simulink model "QuadrupedURDF"  (R2023b)
settings: Solver=VariableStepAuto  StartTime=0.0  StopTime=10.0  RelTol=1e-3
undefined symbols (not defined in the file or in its folder): body_mass, desired_speed, equilibrium_length, fixed_time, k_landing_angle, k_slip, kd, kp, lower_leg_length, max_torque, shin_mass, thigh_mass, upper_leg_length, X, x_contact, Y, y_contact, Z, z_contact
libraries: sm_lib x94, nesl_utility x21, slpidlib x10
(part 3 of 3)

== system QuadrupedURDF/Environment//Plant/Rear_Right_Thigh ==
  Inertia : sm_lib/Body Elements/Inertia  InertiaType=Custom  Mass=thigh_mass  MassUnits=kg  CenterOfMass=[0, 0, 0]  CenterOfMassUnits=m  MomentsOfInertia=[0.000703443703532356, 0.000379089863098611, 0.00102411507237722]  MomentsOfInertiaUnits=kg*m^2  ProductsOfInertia=[-1.02974442751944e-06, -1.25476848652012e-07, 5.05069776933996e-07]  ProductsOfInertiaUnits=kg*m^2  GraphicType=None  MarkerShape=Inertia  MarkerSize=20  GraphicVisPropType=SimpleVisualProperties  GraphicDiffuseColor=[0.5 0.5 0.5]  GraphicSpecularColor=[0.5 0.5 0.5 1.0]  GraphicAmbientColor=[0.15 0.15 0.15 1.0]  GraphicEmissiveColor=[0.0 0.0 0.0 1.0]  GraphicShininess=75  GraphicOpacity=1.0
  InertiaOriginTransform : sm_lib/Frames and Transforms/Rigid Transform  TranslationMethod=Cartesian  TranslationStandardOffset=0  TranslationStandardOffsetUnits=m  TranslationStandardAxis=+Z  TranslationCartesianOffset=[2.43741414215626e-05, -0.0142051404026354, -0.00547111407205259]  TranslationCartesianOffsetUnits=m  TranslationROffset=0  TranslationROffsetUnits=m  TranslationZOffset=0  TranslationZOffsetUnits=m  TranslationThetaOffset=0  TranslationThetaOffsetUnits=deg  RotationMethod=RotationSequence  RotationAngleUnits=deg  RotationStandardAxis=+Z  RotationAngle=0.0  RotationArbitraryAxis=[0 0 1]  FollAlignAxisA=+X  BaseAlignAxisA=+Y  FollAlignAxisB=+Y  BaseAlignAxisB=+Z  RotationSequenceAxes=BaseAxes  RotationSequence=XYZ  RotationSequenceAngles=[0, 0, 0]  RotationSequenceAnglesUnits=rad  RotationMatrix=[1 0 0; 0 1 0; 0 0 1]  Quaternion=[1 0 0 0]
  Rear_Right_Hip_AxisInvTransform : sm_lib/Frames and Transforms/Rigid Transform  TranslationMethod=Cartesian  TranslationStandardOffset=0  TranslationStandardOffsetUnits=m  TranslationStandardAxis=+Z  TranslationCartesianOffset=[0, 0, 0]  TranslationCartesianOffsetUnits=m  TranslationROffset=0  TranslationROffsetUnits=m  TranslationZOffset=0  TranslationZOffsetUnits=m  TranslationThetaOffset=0  TranslationThetaOffsetUnits=deg  RotationMethod=ArbitraryAxis  RotationAngleUnits=rad  RotationStandardAxis=+Z  RotationAngle=3.141592653589793  RotationArbitraryAxis=[1, 0, 0]  FollAlignAxisA=+X  BaseAlignAxisA=+Y  FollAlignAxisB=+Y  BaseAlignAxisB=+Z  RotationSequenceAxes=FollowerAxes  RotationSequence=XYX  RotationSequenceAngles=[0 0 0]  RotationSequenceAnglesUnits=deg  RotationMatrix=[1 0 0; 0 1 0; 0 0 1]  Quaternion=[1 0 0 0]
  Rear_Right_Knee_AxisTransform : sm_lib/Frames and Transforms/Rigid Transform  TranslationMethod=Cartesian  TranslationStandardOffset=0  TranslationStandardOffsetUnits=m  TranslationStandardAxis=+Z  TranslationCartesianOffset=[0, 0, 0]  TranslationCartesianOffsetUnits=m  TranslationROffset=0  TranslationROffsetUnits=m  TranslationZOffset=0  TranslationZOffsetUnits=m  TranslationThetaOffset=0  TranslationThetaOffsetUnits=deg  RotationMethod=ArbitraryAxis  RotationAngleUnits=rad  RotationStandardAxis=+Z  RotationAngle=0  RotationArbitraryAxis=[1, 0, 0]  FollAlignAxisA=+X  BaseAlignAxisA=+Y  FollAlignAxisB=+Y  BaseAlignAxisB=+Z  RotationSequenceAxes=FollowerAxes  RotationSequence=XYX  RotationSequenceAngles=[0 0 0]  RotationSequenceAnglesUnits=deg  RotationMatrix=[1 0 0; 0 1 0; 0 0 1]  Quaternion=[1 0 0 0]
  Rear_Right_Knee_OriginTransform : sm_lib/Frames and Transforms/Rigid Transform  TranslationMethod=Cartesian  TranslationStandardOffset=0  TranslationStandardOffsetUnits=m  TranslationStandardAxis=+Z  TranslationCartesianOffset=[0, -0.13624999987, 0.0151249999999999]  TranslationCartesianOffsetUnits=m  TranslationROffset=0  TranslationROffsetUnits=m  TranslationZOffset=0  TranslationZOffsetUnits=m  TranslationThetaOffset=0  TranslationThetaOffsetUnits=deg  RotationMethod=RotationSequence  RotationAngleUnits=deg  RotationStandardAxis=+Z  RotationAngle=0.0  RotationArbitraryAxis=[0 0 1]  FollAlignAxisA=+X  BaseAlignAxisA=+Y  FollAlignAxisB=+Y  BaseAlignAxisB=+Z  RotationSequenceAxes=BaseAxes  RotationSequence=XYZ  RotationSequenceAngles=[0, 0, 0]  RotationSequenceAnglesUnits=rad  RotationMatrix=[1 0 0; 0 1 0; 0 0 1]  Quaternion=[1 0 0 0]
  ReferenceFrame : sm_lib/Frames and Transforms/Reference Frame
  Visual : sm_lib/Body Elements/File Solid  ExtGeomFileName=Quadruped URDF/meshes/Rear Right Thigh.STL  UnitType=Custom  ExtGeomFileUnits=m  StepReaderType=HEX  ExportConvexHullGeometry=off  InertiaType=Custom  Mass=0  MassUnits=kg  CenterOfMass=[0, 0, 0]  CenterOfMassUnits=m  MomentsOfInertia=[0, 0, 0]  MomentsOfInertiaUnits=kg*m^2  ProductsOfInertia=[0, 0, 0]  ProductsOfInertiaUnits=kg*m^2  BasedOnType=DensityFromFile  Density=1000  DensityUnits=kg/m^3  DoExposeReferenceFrame=on  SerializedFrames=<Frames/>  GraphicType=FromGeometry  MarkerShape=Sphere  MarkerSize=10  GraphicVisPropType=SimpleVisualProperties  GraphicDiffuseColor=[1, 1, 1]  GraphicSpecularColor=[0.5 0.5 0.5 1.0]  GraphicAmbientColor=[0.15 0.15 0.15 1.0]  GraphicEmissiveColor=[0.0 0.0 0.0 1.0]  GraphicShininess=75  GraphicOpacity=1
  VisualOriginTransform : sm_lib/Frames and Transforms/Rigid Transform  TranslationMethod=Cartesian  TranslationStandardOffset=0  TranslationStandardOffsetUnits=m  TranslationStandardAxis=+Z  TranslationCartesianOffset=[0, 0, 0]  TranslationCartesianOffsetUnits=m  TranslationROffset=0  TranslationROffsetUnits=m  TranslationZOffset=0  TranslationZOffsetUnits=m  TranslationThetaOffset=0  TranslationThetaOffsetUnits=deg  RotationMethod=RotationSequence  RotationAngleUnits=deg  RotationStandardAxis=+Z  RotationAngle=0.0  RotationArbitraryAxis=[0 0 1]  FollAlignAxisA=+X  BaseAlignAxisA=+Y  FollAlignAxisB=+Y  BaseAlignAxisB=+Z  RotationSequenceAxes=BaseAxes  RotationSequence=XYZ  RotationSequenceAngles=[0, 0, 0]  RotationSequenceAnglesUnits=rad  RotationMatrix=[1 0 0; 0 1 0; 0 0 1]  Quaternion=[1 0 0 0]
  F : PMIOPort  Side=Left
  F1 : PMIOPort  Port=2  Side=Right
  connections:
  Inertia/RConn1 -- InertiaOriginTransform/RConn1
  Rear_Right_Hip_AxisInvTransform/RConn1 -- F/RConn1
  Rear_Right_Knee_AxisTransform/RConn1 -- F1/RConn1
  Rear_Right_Knee_AxisTransform/LConn1 -- Rear_Right_Knee_OriginTransform/RConn1
  Rear_Right_Hip_AxisInvTransform/LConn1 -- InertiaOriginTransform/LConn1 -- ReferenceFrame/RConn1 -- VisualOriginTransform/LConn1 -- Rear_Right_Knee_OriginTransform/LConn1
  Visual/RConn1 -- VisualOriginTransform/RConn1

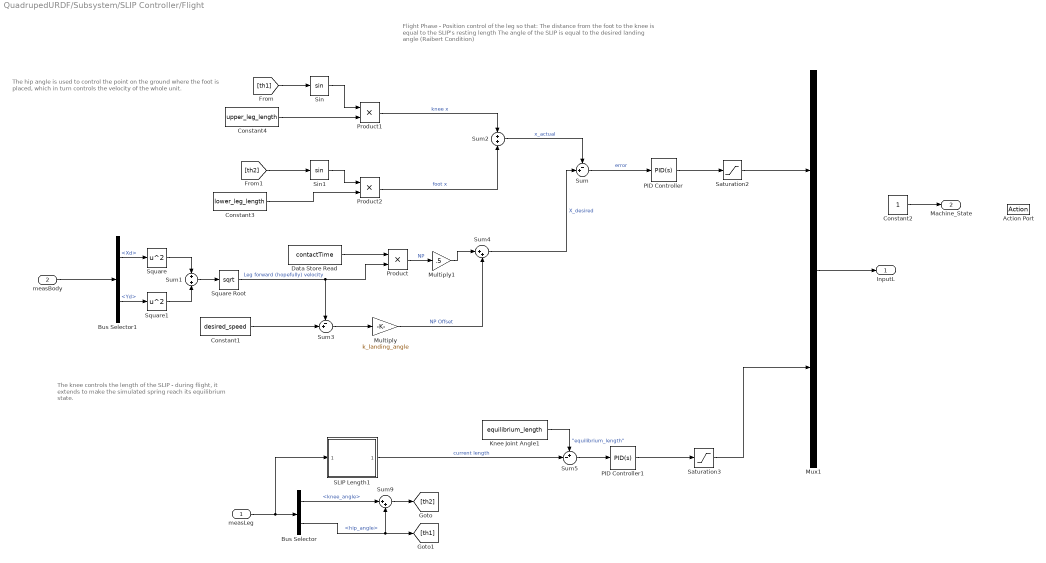
== system QuadrupedURDF/Subsystem/SLIP Controller/Flight ==
  note: Flight Phase - Position control of the leg so that:
      | The distance from the foot to the knee is equal to the SLIP's resting length
      | The angle of the SLIP is equal to the desired landing angle (Raibert Condition)
  note: The hip angle is used to control the point on the ground where the foot is
      | placed, which in turn controls the velocity of the whole unit.
  note: The knee controls the length of the SLIP - during flight, it
      | extends to make the simulated spring reach its equilibrium
      | state.
  measLeg : Inport
  measBody : Inport  Port=2
  Action Port : ActionPort
      settings: CopyFcn=Stateflow.SLINSF.SimulinkMan.removeBlockPreDeleteFcn  PreDeleteFcn=Stateflow.SLINSF.SimulinkMan.unsafePredeleteFcn
  Bus Selector : BusSelector  OutputSignals=knee_angle,hip_angle
  Bus Selector1 : BusSelector  OutputSignals=Xd,Yd
  Constant1 : Constant  Value=desired_speed
  Constant2 : Constant
  Constant3 : Constant  Value=lower_leg_length
  Constant4 : Constant  Value=upper_leg_length
  Data Store Read : DataStoreRead  DataStoreName=contactTime  IndexOptions=Index vector (dialog)  Indices=1  OutputSizes=1
  Knee Joint Angle1 : Constant  Value=equilibrium_length
  Multiply : Gain  Gain=k_landing_angle
  Multiply1 : Gain  Gain=.5
  Mux1 : Mux  Inputs=2
  PID Controller : slpidlib/PID Controller  Controller=PID  Form=Parallel  TimeDomain=Continuous-time  UseExternalTs=off  SampleTime=-1  IntegratorMethod=Forward Euler  FilterMethod=Forward Euler  ControllerParametersSource=internal  P=50  I=0  UseKiTs=off  D=10  N=100  UseFilter=on  TunerSelectOption=Transfer Function Based (PID Tuner App)  InitialConditionSource=internal  InitialConditionForIntegrator=0  InitialConditionForFilter=0  DifferentiatorICPrevScaledInput=0  ExternalReset=none  TrackingMode=off  Kt=1  LimitOutput=off  SatLimitsSource=internal  UpperSaturationLimit=inf  LowerSaturationLimit=-inf  LinearizeAsGain=on  AntiWindupMode=none  Kb=1  LimitIntegrator=off  UpperIntegratorSaturationLimit=inf  LowerIntegratorSaturationLimit=-inf  POutMin=[]  POutMax=[]  IOutMin=[]  IOutMax=[]  DOutMin=[]  DOutMax=[]  NOutMin=[]  NOutMax=[]  SumOutMin=[]  SumOutMax=[]  SaturationOutMin=[]  SaturationOutMax=[]  PParamMin=[]  PParamMax=[]  IParamMin=[]  IParamMax=[]  DParamMin=[]  DParamMax=[]  NParamMin=[]  NParamMax=[]  KbParamMin=[]  KbParamMax=[]  KtParamMin=[]  KtParamMax=[]  KbOutMin=[]  KbOutMax=[]  KtOutMin=[]  KtOutMax=[]  IntegratorOutMin=[]  IntegratorOutMax=[]  FilterOutMin=[]  FilterOutMax=[]  SumI1OutMin=[]  SumI1OutMax=[]  SumI2OutMin=[]  SumI2OutMax=[]  SumI3OutMin=[]  SumI3OutMax=[]  SumI4OutMin=[]  SumI4OutMax=[]  SumDOutMin=[]  SumDOutMax=[]  DifferentiatorOutMin=[]  DifferentiatorOutMax=[]  FilterDiffOutCoefMin=[]  FilterDiffOutCoefMax=[]  ReciprocalOutMin=[]  ReciprocalOutMax=[]  SumDenOutMin=[]  SumDenOutMax=[]  SumNumOutMin=[]  SumNumOutMax=[]  DivideOutMin=[]  DivideOutMax=[]  UdiffTsProdOutMin=[]  UdiffTsProdOutMax=[]  NTsProdOutMin=[]  NTsProdOutMax=[]  UintegralTsProdOutMin=[]  UintegralTsProdOutMax=[]  UngainTsProdOutMin=[]  UngainTsProdOutMax=[]  ClampingZeroOutDataTypeStr=Inherit: Inherit via back propagation  ClampingZeroOutMin=[]  ClampingZeroOutMax=[]  FilterDenConstantOutDataTypeStr=Inherit: Inherit via back propagation  FilterDenConstantOutMin=[]  FilterDenConstantOutMax=[]  PCopyOutDataTypeStr=Inherit: Inherit via back propagation  PCopyOutMin=[]  PCopyOutMax=[]  NCopyOutDataTypeStr=Inherit: Inherit via back propagation  NCopyOutMin=[]  NCopyOutMax=[]  IntegratorContinuousStateAttributes=''  IntegratorStateMustResolveToSignalObject=off  IntegratorRTWStateStorageClass=Auto  FilterContinuousStateAttributes=''  FilterStateMustResolveToSignalObject=off  FilterRTWStateStorageClass=Auto  ParallelPVariant=InternalParameters  IdealPVariant=Disabled  IVariant=InternalParameters  DVariant=InternalParameters  IntegratorVariant=Continuous  SatVariant=Disabled  AWVariant=Passthrough  PCopyVariant=Disabled  TRVariant=Disabled  FdbkBlocksVariant=Forward  IdealPFdbkVariant=Disabled  SatFdbkVariant=Disabled  DerivativeFilterVariant=ContFilter  NVariant=InternalParameters  NCopyVariant=Disabled  FilterICVariant=InternalICsFilter  IntegratorICVariant=InternalICs  ExternalResetVariant=Disabled  TRSumVariant=Passthrough  SumFdbkVariant=Disabled  SumVariant=Sum_PID  TsampFilterVariant=InternalTs  TsampNgainVariant=Passthrough  TsampIntegralVariant=Disabled_SignalSpec  ExternalSaturationOutDataTypeStr=Inherit: Same as second input
  PID Controller1 : slpidlib/PID Controller  Controller=PID  Form=Parallel  TimeDomain=Continuous-time  UseExternalTs=off  SampleTime=-1  IntegratorMethod=Forward Euler  FilterMethod=Forward Euler  ControllerParametersSource=internal  P=50  I=0  UseKiTs=off  D=5  N=100  UseFilter=on  TunerSelectOption=Transfer Function Based (PID Tuner App)  InitialConditionSource=internal  InitialConditionForIntegrator=0  InitialConditionForFilter=0  DifferentiatorICPrevScaledInput=0  ExternalReset=none  TrackingMode=off  Kt=1  LimitOutput=off  SatLimitsSource=internal  UpperSaturationLimit=inf  LowerSaturationLimit=-inf  LinearizeAsGain=on  AntiWindupMode=none  Kb=1  LimitIntegrator=off  UpperIntegratorSaturationLimit=inf  LowerIntegratorSaturationLimit=-inf  POutMin=[]  POutMax=[]  IOutMin=[]  IOutMax=[]  DOutMin=[]  DOutMax=[]  NOutMin=[]  NOutMax=[]  SumOutMin=[]  SumOutMax=[]  SaturationOutMin=[]  SaturationOutMax=[]  PParamMin=[]  PParamMax=[]  IParamMin=[]  IParamMax=[]  DParamMin=[]  DParamMax=[]  NParamMin=[]  NParamMax=[]  KbParamMin=[]  KbParamMax=[]  KtParamMin=[]  KtParamMax=[]  KbOutMin=[]  KbOutMax=[]  KtOutMin=[]  KtOutMax=[]  IntegratorOutMin=[]  IntegratorOutMax=[]  FilterOutMin=[]  FilterOutMax=[]  SumI1OutMin=[]  SumI1OutMax=[]  SumI2OutMin=[]  SumI2OutMax=[]  SumI3OutMin=[]  SumI3OutMax=[]  SumI4OutMin=[]  SumI4OutMax=[]  SumDOutMin=[]  SumDOutMax=[]  DifferentiatorOutMin=[]  DifferentiatorOutMax=[]  FilterDiffOutCoefMin=[]  FilterDiffOutCoefMax=[]  ReciprocalOutMin=[]  ReciprocalOutMax=[]  SumDenOutMin=[]  SumDenOutMax=[]  SumNumOutMin=[]  SumNumOutMax=[]  DivideOutMin=[]  DivideOutMax=[]  UdiffTsProdOutMin=[]  UdiffTsProdOutMax=[]  NTsProdOutMin=[]  NTsProdOutMax=[]  UintegralTsProdOutMin=[]  UintegralTsProdOutMax=[]  UngainTsProdOutMin=[]  UngainTsProdOutMax=[]  ClampingZeroOutDataTypeStr=Inherit: Inherit via back propagation  ClampingZeroOutMin=[]  ClampingZeroOutMax=[]  FilterDenConstantOutDataTypeStr=Inherit: Inherit via back propagation  FilterDenConstantOutMin=[]  FilterDenConstantOutMax=[]  PCopyOutDataTypeStr=Inherit: Inherit via back propagation  PCopyOutMin=[]  PCopyOutMax=[]  NCopyOutDataTypeStr=Inherit: Inherit via back propagation  NCopyOutMin=[]  NCopyOutMax=[]  IntegratorContinuousStateAttributes=''  IntegratorStateMustResolveToSignalObject=off  IntegratorRTWStateStorageClass=Auto  FilterContinuousStateAttributes=''  FilterStateMustResolveToSignalObject=off  FilterRTWStateStorageClass=Auto  ParallelPVariant=InternalParameters  IdealPVariant=Disabled  IVariant=InternalParameters  DVariant=InternalParameters  IntegratorVariant=Continuous  SatVariant=Disabled  AWVariant=Passthrough  PCopyVariant=Disabled  TRVariant=Disabled  FdbkBlocksVariant=Forward  IdealPFdbkVariant=Disabled  SatFdbkVariant=Disabled  DerivativeFilterVariant=ContFilter  NVariant=InternalParameters  NCopyVariant=Disabled  FilterICVariant=InternalICsFilter  IntegratorICVariant=InternalICs  ExternalResetVariant=Disabled  TRSumVariant=Passthrough  SumFdbkVariant=Disabled  SumVariant=Sum_PID  TsampFilterVariant=InternalTs  TsampNgainVariant=Passthrough  TsampIntegralVariant=Disabled_SignalSpec  ExternalSaturationOutDataTypeStr=Inherit: Same as second input
  Product : Product
  Product1 : Product
  Product2 : Product
  SLIP Length1 : Subsystem
  Saturation2 : Saturate  UpperLimit=max_torque  LowerLimit=-max_torque
  Saturation3 : Saturate  UpperLimit=max_torque  LowerLimit=-max_torque
  Sin : Trigonometry
  Sin1 : Trigonometry
  Square : Math  Operator=square
  Square Root : Sqrt
  Square1 : Math  Operator=square
  Sum : Sum  Inputs=-+|
  Sum1 : Sum  Inputs=+|+
  Sum2 : Sum  Inputs=+|+
  Sum3 : Sum  Inputs=-+|
  Sum4 : Sum  Inputs=|++
  Sum5 : Sum  Inputs=+-|
  Sum9 : Sum  Inputs=|++
  InputL : Outport
  Machine_State : Outport  Port=2
  wires:
  Sum1/1 -> Square Root/1
  Bus Selector1/2 -> Square1/1  "<Yd>"
  Product1/1 -> Sum2/1  "knee x"
  Sin1/1 -> Product2/1
  [th1] -> Sin/1
  Constant2/1 -> Machine_State/1
  Saturation3/1 -> Mux1/2
  Sum4/1 -> Sum/2  "X_desired"
  Knee Joint Angle1/1 -> Sum5/1  "\"equilibrium_length\""
  Multiply1/1 -> Sum4/1
  Constant1/1 -> Sum3/2
  Sin/1 -> Product1/1
  [th2] -> Sin1/1
  Sum5/1 -> PID Controller1/1
  PID Controller/1 -> Saturation2/1
  Bus Selector1/1 -> Square/1  "<Xd>"
  Data Store Read/1 -> Product/1
  Bus Selector/2 -> Sum9/2, [th1]  "<hip_angle>"
  Multiply/1 -> Sum4/2  "NP Offset"
  Sum9/1 -> [th2]
  Bus Selector/1 -> Sum9/1  "<knee_angle>"
  measLeg/1 -> SLIP Length1/1(measLeg), Bus Selector/1
  SLIP Length1/1(current length) -> Sum5/2  "current length"
  Square Root/1 -> Product/2, Sum3/1  "Leg forward (hopefully) velocity"
  PID Controller1/1 -> Saturation3/1
  Sum3/1 -> Multiply/1
  Saturation2/1 -> Mux1/1
  Mux1/1 -> InputL/1
  Constant4/1 -> Product1/2
  Sum/1 -> PID Controller/1  "error"
  Sum2/1 -> Sum/1  "x_actual"
  Product2/1 -> Sum2/2  "foot x"
  Product/1 -> Multiply1/1  "NP"
  Constant3/1 -> Product2/2
  Square1/1 -> Sum1/2
  Square/1 -> Sum1/1
  measBody/1 -> Bus Selector1/1

== system QuadrupedURDF/Subsystem/SLIP Controller/Stance ==
  note: Stance Phase - the SLIP is allowed to dictate the reaction of the leg
  measLeg : Inport
  Action Port : ActionPort
      settings: CopyFcn=Stateflow.SLINSF.SimulinkMan.removeBlockPreDeleteFcn  PreDeleteFcn=Stateflow.SLINSF.SimulinkMan.unsafePredeleteFcn
  Constant2 : Constant  Value=3
  Hip Torque Calculation : Subsystem
  Knee Torque Calculation : Subsystem
  Mux : Mux  Inputs=2
  Saturation : Saturate  UpperLimit=max_torque  LowerLimit=-max_torque
  Saturation1 : Saturate  UpperLimit=max_torque  LowerLimit=-max_torque
  InputL : Outport
  Machine_State : Outport  Port=2
  wires:
  Mux/1 -> InputL/1
  Constant2/1 -> Machine_State/1
  Knee Torque Calculation/1(knee torque) -> Saturation1/1  "knee torque unsat"
  Saturation/1 -> Mux/1  "hip torque sat"
  Saturation1/1 -> Mux/2  "knee torque sat"
  Hip Torque Calculation/1(hip torque) -> Knee Torque Calculation/1(hip torque), Saturation/1  "hip torque unsat"
  measLeg/1 -> Hip Torque Calculation/1(measLeg), Knee Torque Calculation/2(measLeg)

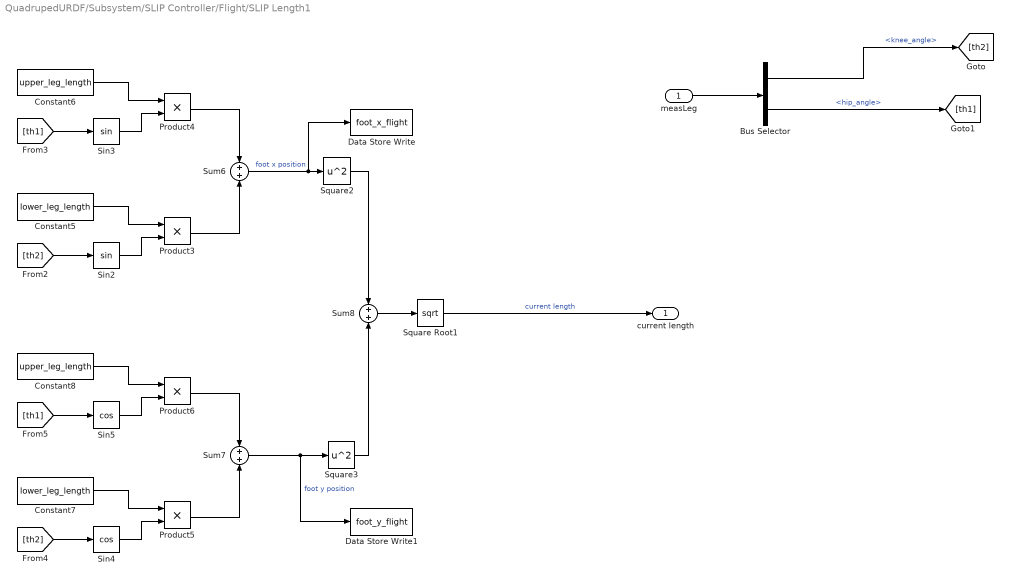
== system QuadrupedURDF/Subsystem/SLIP Controller/Flight/SLIP Length1 ==
  measLeg : Inport
  Bus Selector : BusSelector  OutputSignals=knee_angle,hip_angle
  Constant5 : Constant  Value=lower_leg_length
  Constant6 : Constant  Value=upper_leg_length
  Constant7 : Constant  Value=lower_leg_length
  Constant8 : Constant  Value=upper_leg_length
  Data Store Write : DataStoreWrite  DataStoreName=foot_x_flight  IndexOptions=Index vector (dialog)  Indices=1  OutputSizes=1
  Data Store Write1 : DataStoreWrite  DataStoreName=foot_y_flight  IndexOptions=Index vector (dialog)  Indices=1  OutputSizes=1
  Product{3..6} (4 alike) : Product
  Sin2 : Trigonometry
  Sin3 : Trigonometry
  Sin4 : Trigonometry  Operator=cos
  Sin5 : Trigonometry  Operator=cos
  Square Root1 : Sqrt
  Square2 : Math  Operator=square
  Square3 : Math  Operator=square
  Sum6 : Sum  Inputs=+|+
  Sum7 : Sum  Inputs=+|+
  Sum8 : Sum  Inputs=+|+
  current length : Outport
  wires:
  Square2/1 -> Sum8/1
  Sum7/1 -> Data Store Write1/1, Square3/1  "foot y position"
  [th2] -> Sin2/1
  Square3/1 -> Sum8/2
  Sin4/1 -> Product5/2
  Constant5/1 -> Product3/1
  Constant7/1 -> Product5/1
  Product6/1 -> Sum7/1
  Product3/1 -> Sum6/2
  [th2] -> Sin4/1
  Product5/1 -> Sum7/2
  [th1] -> Sin5/1
  Sin3/1 -> Product4/2
  Constant8/1 -> Product6/1
  Sin5/1 -> Product6/2
  Sin2/1 -> Product3/2
  Sum6/1 -> Data Store Write/1, Square2/1  "foot x position"
  Constant6/1 -> Product4/1
  Product4/1 -> Sum6/1
  Sum8/1 -> Square Root1/1
  [th1] -> Sin3/1
  Square Root1/1 -> current length/1  "current length"
  Bus Selector/1 -> [th2]  "<knee_angle>"
  Bus Selector/2 -> [th1]  "<hip_angle>"
  measLeg/1 -> Bus Selector/1

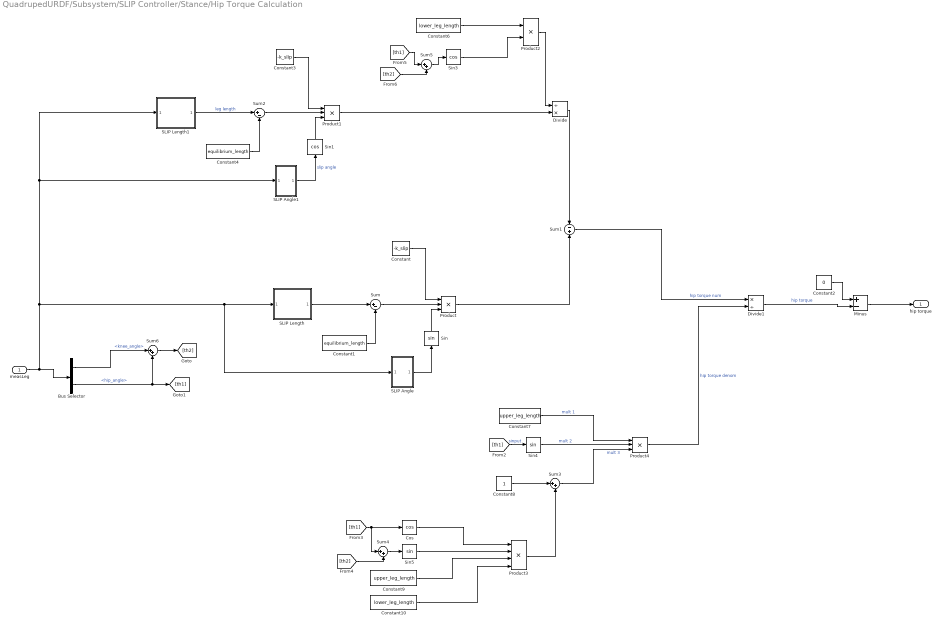
== system QuadrupedURDF/Subsystem/SLIP Controller/Stance/Hip Torque Calculation ==
  measLeg : Inport
  Bus Selector : BusSelector  OutputSignals=knee_angle,hip_angle
  Constant : Constant  Value=-k_slip
  Constant1 : Constant  Value=equilibrium_length
  Constant10 : Constant  Value=lower_leg_length
  Constant2 : Constant  Value=0
  Constant3 : Constant  Value=-k_slip
  Constant4 : Constant  Value=equilibrium_length
  Constant6 : Constant  Value=lower_leg_length
  Constant7 : Constant  Value=upper_leg_length
  Constant8 : Constant
  Constant9 : Constant  Value=upper_leg_length
  Cos : Trigonometry  Operator=cos
  Divide : Product  Inputs=/*
  Divide1 : Product  Inputs=*/
  Minus : Sum  Inputs=+-
  Product : Product  Inputs=3
  Product1 : Product  Inputs=3
  Product2 : Product
  Product3 : Product  Inputs=4
  Product4 : Product  Inputs=3
  SLIP Angle : Subsystem
  SLIP Angle1 : Subsystem
  SLIP Length : Subsystem
  SLIP Length1 : Subsystem
  Sin : Trigonometry
  Sin1 : Trigonometry  Operator=cos
  Sin3 : Trigonometry  Operator=cos
  Sin4 : Trigonometry
  Sin5 : Trigonometry
  Sum : Sum  Inputs=|+-
  Sum1 : Sum  Inputs=-|+
  Sum2 : Sum  Inputs=|+-
  Sum{3..6} (4 alike) : Sum  Inputs=|++
  hip torque : Outport
  wires:
  Sin1/1 -> Product1/3
  [th2] -> Sum4/2
  Constant/1 -> Product/1
  Sin5/1 -> Product3/2
  Constant7/1 -> Product4/1  "mult 1"
  Constant1/1 -> Sum/2
  Product2/1 -> Divide/1
  Product/1 -> Sum1/2
  Sin/1 -> Product/3
  Constant6/1 -> Product2/1
  Constant9/1 -> Product3/3
  Sum/1 -> Product/2
  Product3/1 -> Sum3/2
  Constant10/1 -> Product3/4
  SLIP Angle/1(Out1) -> Sin/1
  Sum1/1 -> Divide1/1  "hip torque num"
  Sum2/1 -> Product1/2
  Product4/1 -> Divide1/2  "hip torque denom"
  SLIP Length1/1(current length) -> Sum2/1  "leg length"
  Constant4/1 -> Sum2/2
  SLIP Angle1/1(Out1) -> Sin1/1  "slip angle"
  Divide1/1 -> Minus/2  "hip torque"
  Constant3/1 -> Product1/1
  Product1/1 -> Divide/2
  [th1] -> Sum4/1, Cos/1
  Sin3/1 -> Product2/2
  Sin4/1 -> Product4/2  "mult 2"
  Divide/1 -> Sum1/1
  SLIP Length/1(current length) -> Sum/1
  Sum3/1 -> Product4/3  "mult 3"
  [th1] -> Sin4/1  "sinput"
  Constant8/1 -> Sum3/1
  Cos/1 -> Product3/1
  Constant2/1 -> Minus/1
  Minus/1 -> hip torque/1
  Sum4/1 -> Sin5/1
  [th1] -> Sum5/1
  [th2] -> Sum5/2
  Sum5/1 -> Sin3/1
  measLeg/1 -> Bus Selector/1, SLIP Angle/1(measLeg), SLIP Length/1(measLeg), SLIP Angle1/1(measLeg), SLIP Length1/1(measLeg)
  Bus Selector/1 -> Sum6/1  "<knee_angle>"
  Bus Selector/2 -> Sum6/2, [th1]  "<hip_angle>"
  Sum6/1 -> [th2]

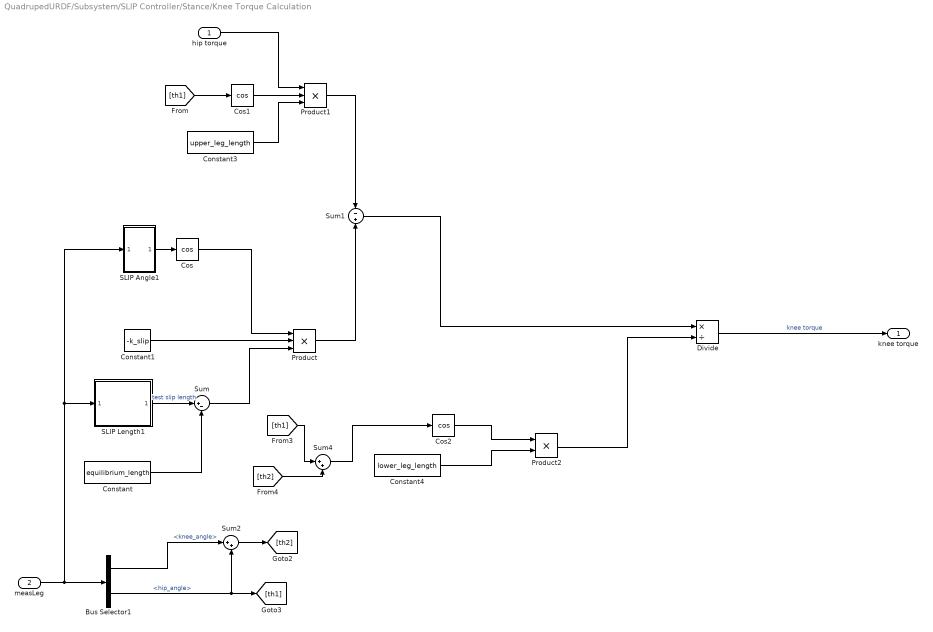
== system QuadrupedURDF/Subsystem/SLIP Controller/Stance/Knee Torque Calculation ==
  hip torque : Inport
  measLeg : Inport  Port=2
  Bus Selector1 : BusSelector  OutputSignals=knee_angle,hip_angle
  Constant : Constant  Value=equilibrium_length
  Constant1 : Constant  Value=-k_slip
  Constant3 : Constant  Value=upper_leg_length
  Constant4 : Constant  Value=lower_leg_length
  Cos : Trigonometry  Operator=cos
  Cos1 : Trigonometry  Operator=cos
  Cos2 : Trigonometry  Operator=cos
  Divide : Product  Inputs=*/
  Product : Product  Inputs=3
  Product1 : Product  Inputs=3
  Product2 : Product
  SLIP Angle1 : Subsystem
  SLIP Length1 : Subsystem
  Sum : Sum  Inputs=|+-
  Sum1 : Sum  Inputs=-|+
  Sum2 : Sum  Inputs=|++
  Sum4 : Sum  Inputs=|++
  knee torque : Outport
  wires:
  Constant3/1 -> Product1/3
  Constant/1 -> Sum/2
  Cos/1 -> Product/1
  Cos2/1 -> Product2/1
  SLIP Length1/1(current length) -> Sum/1  "test slip length"
  Sum1/1 -> Divide/1
  Constant4/1 -> Product2/2
  Product1/1 -> Sum1/1
  Constant1/1 -> Product/2
  [th1] -> Cos1/1
  Sum4/1 -> Cos2/1
  Cos1/1 -> Product1/2
  Product/1 -> Sum1/2
  SLIP Angle1/1(Out1) -> Cos/1
  Sum/1 -> Product/3
  Product2/1 -> Divide/2
  Divide/1 -> knee torque/1  "knee torque"
  hip torque/1 -> Product1/1
  [th1] -> Sum4/1
  [th2] -> Sum4/2
  measLeg/1 -> Bus Selector1/1, SLIP Length1/1(measLeg), SLIP Angle1/1(measLeg)
  Bus Selector1/1 -> Sum2/1  "<knee_angle>"
  Bus Selector1/2 -> Sum2/2, [th1]  "<hip_angle>"
  Sum2/1 -> [th2]

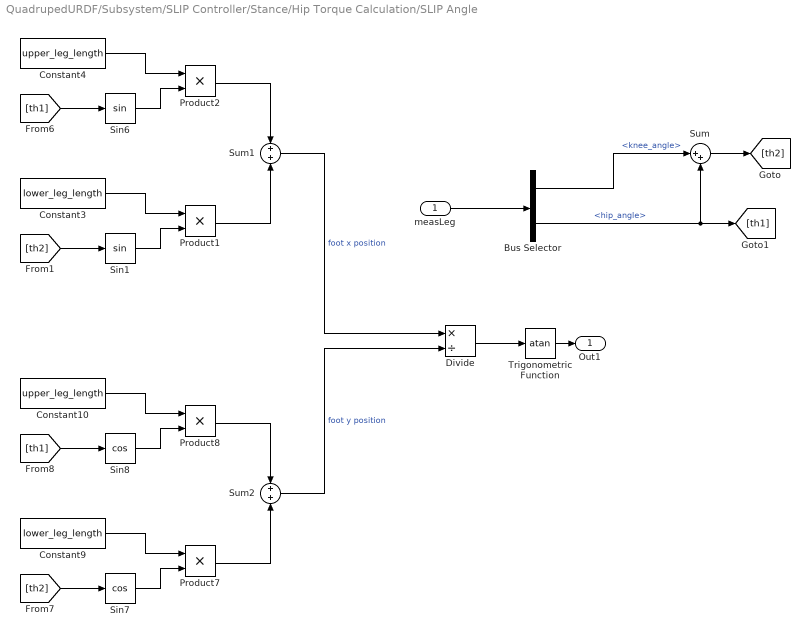
== system QuadrupedURDF/Subsystem/SLIP Controller/Stance/Hip Torque Calculation/SLIP Angle ==
  measLeg : Inport
  Bus Selector : BusSelector  OutputSignals=knee_angle,hip_angle
  Constant10 : Constant  Value=upper_leg_length
  Constant3 : Constant  Value=lower_leg_length
  Constant4 : Constant  Value=upper_leg_length
  Constant9 : Constant  Value=lower_leg_length
  Divide : Product  Inputs=*/
  Product{1..2,7..8} (4 alike) : Product
  Sin1 : Trigonometry
  Sin6 : Trigonometry
  Sin7 : Trigonometry  Operator=cos
  Sin8 : Trigonometry  Operator=cos
  Sum : Sum  Inputs=|++
  Sum1 : Sum  Inputs=+|+
  Sum2 : Sum  Inputs=+|+
  Trigonometric Function : Trigonometry  Operator=atan
  Out1 : Outport
  wires:
  Product2/1 -> Sum1/1
  Constant9/1 -> Product7/1
  Sin7/1 -> Product7/2
  Constant10/1 -> Product8/1
  Sin1/1 -> Product1/2
  [th1] -> Sin8/1
  Sin8/1 -> Product8/2
  Product7/1 -> Sum2/2
  [th2] -> Sin7/1
  Sum2/1 -> Divide/2  "foot y position"
  Trigonometric Function/1 -> Out1/1
  Product8/1 -> Sum2/1
  Sum1/1 -> Divide/1  "foot x position"
  Divide/1 -> Trigonometric Function/1
  [th1] -> Sin6/1
  Sin6/1 -> Product2/2
  [th2] -> Sin1/1
  Constant3/1 -> Product1/1
  Constant4/1 -> Product2/1
  Product1/1 -> Sum1/2
  Bus Selector/1 -> Sum/1  "<knee_angle>"
  Bus Selector/2 -> Sum/2, [th1]  "<hip_angle>"
  measLeg/1 -> Bus Selector/1
  Sum/1 -> [th2]

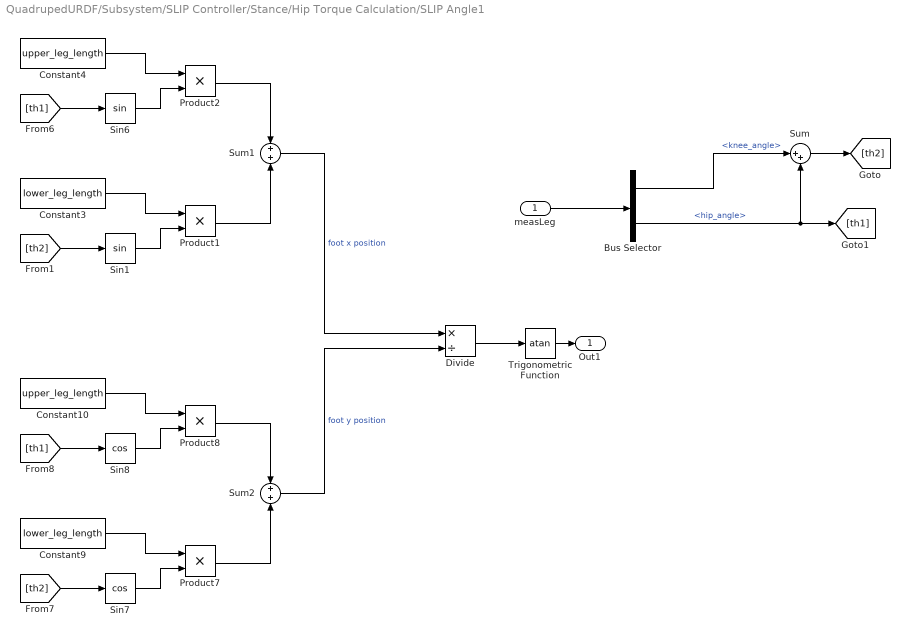
== system QuadrupedURDF/Subsystem/SLIP Controller/Stance/Hip Torque Calculation/SLIP Angle1 ==
  measLeg : Inport
  Bus Selector : BusSelector  OutputSignals=knee_angle,hip_angle
  Constant10 : Constant  Value=upper_leg_length
  Constant3 : Constant  Value=lower_leg_length
  Constant4 : Constant  Value=upper_leg_length
  Constant9 : Constant  Value=lower_leg_length
  Divide : Product  Inputs=*/
  Product{1..2,7..8} (4 alike) : Product
  Sin1 : Trigonometry
  Sin6 : Trigonometry
  Sin7 : Trigonometry  Operator=cos
  Sin8 : Trigonometry  Operator=cos
  Sum : Sum  Inputs=|++
  Sum1 : Sum  Inputs=+|+
  Sum2 : Sum  Inputs=+|+
  Trigonometric Function : Trigonometry  Operator=atan
  Out1 : Outport
  wires:
  Product2/1 -> Sum1/1
  Constant9/1 -> Product7/1
  Sin7/1 -> Product7/2
  Constant10/1 -> Product8/1
  Sin1/1 -> Product1/2
  [th1] -> Sin8/1
  Sin8/1 -> Product8/2
  Product7/1 -> Sum2/2
  [th2] -> Sin7/1
  Sum2/1 -> Divide/2  "foot y position"
  Trigonometric Function/1 -> Out1/1
  Product8/1 -> Sum2/1
  Sum1/1 -> Divide/1  "foot x position"
  Divide/1 -> Trigonometric Function/1
  [th1] -> Sin6/1
  Sin6/1 -> Product2/2
  [th2] -> Sin1/1
  Constant3/1 -> Product1/1
  Constant4/1 -> Product2/1
  Product1/1 -> Sum1/2
  Bus Selector/1 -> Sum/1  "<knee_angle>"
  Bus Selector/2 -> Sum/2, [th1]  "<hip_angle>"
  measLeg/1 -> Bus Selector/1
  Sum/1 -> [th2]

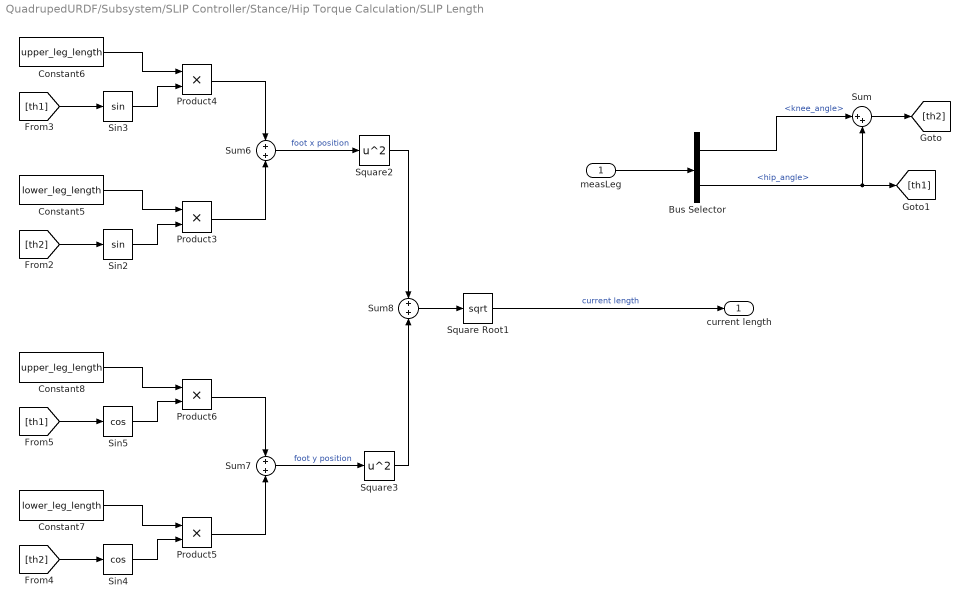
== system QuadrupedURDF/Subsystem/SLIP Controller/Stance/Hip Torque Calculation/SLIP Length ==
  measLeg : Inport
  Bus Selector : BusSelector  OutputSignals=knee_angle,hip_angle
  Constant5 : Constant  Value=lower_leg_length
  Constant6 : Constant  Value=upper_leg_length
  Constant7 : Constant  Value=lower_leg_length
  Constant8 : Constant  Value=upper_leg_length
  Product{3..6} (4 alike) : Product
  Sin2 : Trigonometry
  Sin3 : Trigonometry
  Sin4 : Trigonometry  Operator=cos
  Sin5 : Trigonometry  Operator=cos
  Square Root1 : Sqrt
  Square2 : Math  Operator=square
  Square3 : Math  Operator=square
  Sum : Sum  Inputs=|++
  Sum6 : Sum  Inputs=+|+
  Sum7 : Sum  Inputs=+|+
  Sum8 : Sum  Inputs=+|+
  current length : Outport
  wires:
  Square2/1 -> Sum8/1
  Sum7/1 -> Square3/1  "foot y position"
  [th2] -> Sin2/1
  Square3/1 -> Sum8/2
  Sin4/1 -> Product5/2
  Constant5/1 -> Product3/1
  Constant7/1 -> Product5/1
  Product6/1 -> Sum7/1
  Product3/1 -> Sum6/2
  [th2] -> Sin4/1
  Product5/1 -> Sum7/2
  [th1] -> Sin5/1
  Sin3/1 -> Product4/2
  Constant8/1 -> Product6/1
  Sin5/1 -> Product6/2
  Sin2/1 -> Product3/2
  Sum6/1 -> Square2/1  "foot x position"
  Constant6/1 -> Product4/1
  Product4/1 -> Sum6/1
  Sum8/1 -> Square Root1/1
  [th1] -> Sin3/1
  Square Root1/1 -> current length/1  "current length"
  Bus Selector/1 -> Sum/1  "<knee_angle>"
  Bus Selector/2 -> Sum/2, [th1]  "<hip_angle>"
  measLeg/1 -> Bus Selector/1
  Sum/1 -> [th2]

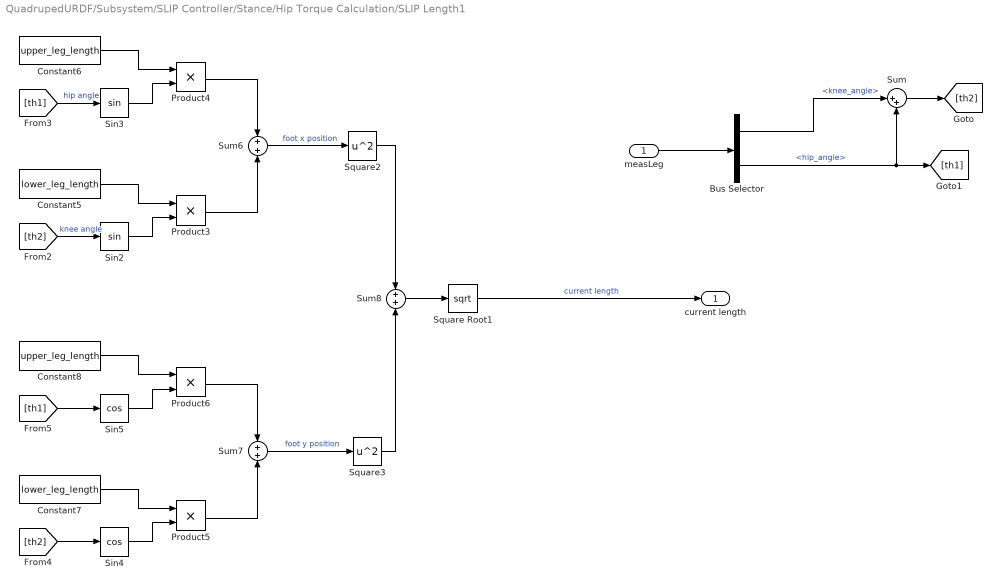
== system QuadrupedURDF/Subsystem/SLIP Controller/Stance/Hip Torque Calculation/SLIP Length1 ==
  measLeg : Inport
  Bus Selector : BusSelector  OutputSignals=knee_angle,hip_angle
  Constant5 : Constant  Value=lower_leg_length
  Constant6 : Constant  Value=upper_leg_length
  Constant7 : Constant  Value=lower_leg_length
  Constant8 : Constant  Value=upper_leg_length
  Product{3..6} (4 alike) : Product
  Sin2 : Trigonometry
  Sin3 : Trigonometry
  Sin4 : Trigonometry  Operator=cos
  Sin5 : Trigonometry  Operator=cos
  Square Root1 : Sqrt
  Square2 : Math  Operator=square
  Square3 : Math  Operator=square
  Sum : Sum  Inputs=|++
  Sum6 : Sum  Inputs=+|+
  Sum7 : Sum  Inputs=+|+
  Sum8 : Sum  Inputs=+|+
  current length : Outport
  wires:
  Square2/1 -> Sum8/1
  Sum7/1 -> Square3/1  "foot y position"
  [th2] -> Sin2/1  "knee angle"
  Square3/1 -> Sum8/2
  Sin4/1 -> Product5/2
  Constant5/1 -> Product3/1
  Constant7/1 -> Product5/1
  Product6/1 -> Sum7/1
  Product3/1 -> Sum6/2
  [th2] -> Sin4/1
  Product5/1 -> Sum7/2
  [th1] -> Sin5/1
  Sin3/1 -> Product4/2
  Constant8/1 -> Product6/1
  Sin5/1 -> Product6/2
  Sin2/1 -> Product3/2
  Sum6/1 -> Square2/1  "foot x position"
  Constant6/1 -> Product4/1
  Product4/1 -> Sum6/1
  Sum8/1 -> Square Root1/1
  [th1] -> Sin3/1  "hip angle"
  Square Root1/1 -> current length/1  "current length"
  Bus Selector/2 -> Sum/2, [th1]  "<hip_angle>"
  measLeg/1 -> Bus Selector/1
  Bus Selector/1 -> Sum/1  "<knee_angle>"
  Sum/1 -> [th2]

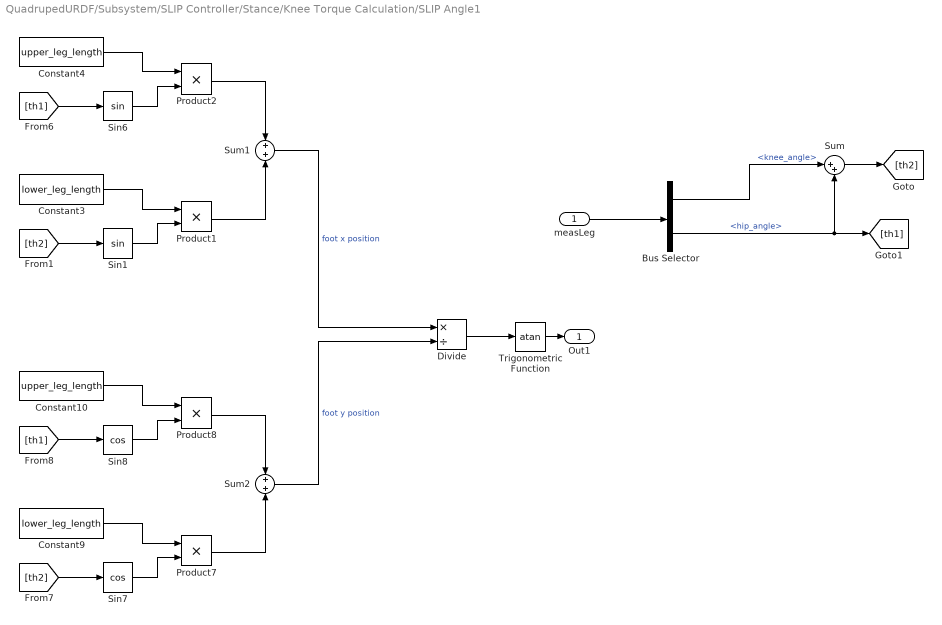
== system QuadrupedURDF/Subsystem/SLIP Controller/Stance/Knee Torque Calculation/SLIP Angle1 ==
  measLeg : Inport
  Bus Selector : BusSelector  OutputSignals=knee_angle,hip_angle
  Constant10 : Constant  Value=upper_leg_length
  Constant3 : Constant  Value=lower_leg_length
  Constant4 : Constant  Value=upper_leg_length
  Constant9 : Constant  Value=lower_leg_length
  Divide : Product  Inputs=*/
  Product{1..2,7..8} (4 alike) : Product
  Sin1 : Trigonometry
  Sin6 : Trigonometry
  Sin7 : Trigonometry  Operator=cos
  Sin8 : Trigonometry  Operator=cos
  Sum : Sum  Inputs=|++
  Sum1 : Sum  Inputs=+|+
  Sum2 : Sum  Inputs=+|+
  Trigonometric Function : Trigonometry  Operator=atan
  Out1 : Outport
  wires:
  Product2/1 -> Sum1/1
  Constant9/1 -> Product7/1
  Sin7/1 -> Product7/2
  Constant10/1 -> Product8/1
  Sin1/1 -> Product1/2
  [th1] -> Sin8/1
  Sin8/1 -> Product8/2
  Product7/1 -> Sum2/2
  [th2] -> Sin7/1
  Sum2/1 -> Divide/2  "foot y position"
  Trigonometric Function/1 -> Out1/1
  Product8/1 -> Sum2/1
  Sum1/1 -> Divide/1  "foot x position"
  Divide/1 -> Trigonometric Function/1
  [th1] -> Sin6/1
  Sin6/1 -> Product2/2
  [th2] -> Sin1/1
  Constant3/1 -> Product1/1
  Constant4/1 -> Product2/1
  Product1/1 -> Sum1/2
  Bus Selector/1 -> Sum/1  "<knee_angle>"
  Bus Selector/2 -> Sum/2, [th1]  "<hip_angle>"
  measLeg/1 -> Bus Selector/1
  Sum/1 -> [th2]

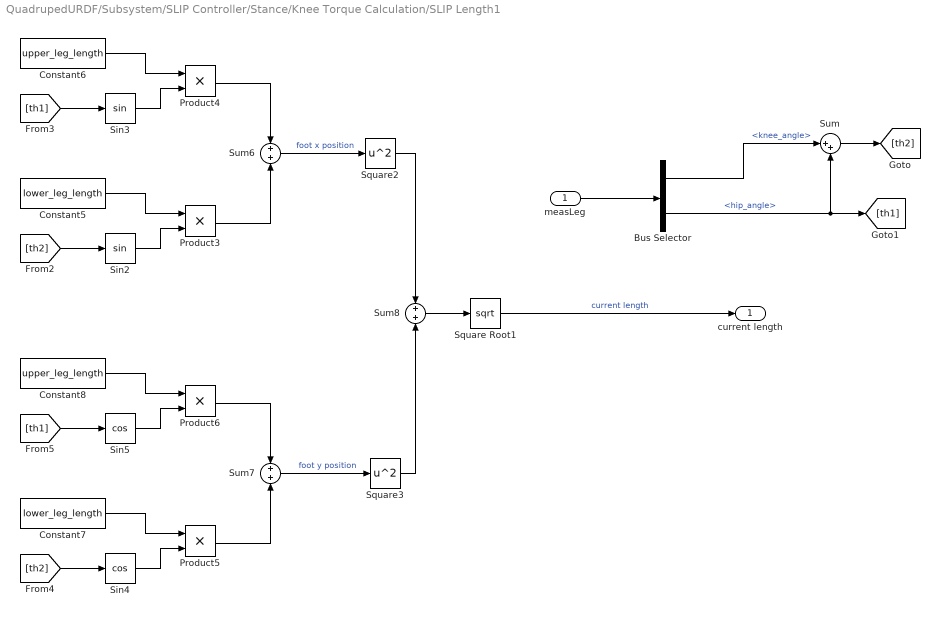
== system QuadrupedURDF/Subsystem/SLIP Controller/Stance/Knee Torque Calculation/SLIP Length1 ==
  measLeg : Inport
  Bus Selector : BusSelector  OutputSignals=knee_angle,hip_angle
  Constant5 : Constant  Value=lower_leg_length
  Constant6 : Constant  Value=upper_leg_length
  Constant7 : Constant  Value=lower_leg_length
  Constant8 : Constant  Value=upper_leg_length
  Product{3..6} (4 alike) : Product
  Sin2 : Trigonometry
  Sin3 : Trigonometry
  Sin4 : Trigonometry  Operator=cos
  Sin5 : Trigonometry  Operator=cos
  Square Root1 : Sqrt
  Square2 : Math  Operator=square
  Square3 : Math  Operator=square
  Sum : Sum  Inputs=|++
  Sum6 : Sum  Inputs=+|+
  Sum7 : Sum  Inputs=+|+
  Sum8 : Sum  Inputs=+|+
  current length : Outport
  wires:
  Square2/1 -> Sum8/1
  Sum7/1 -> Square3/1  "foot y position"
  [th2] -> Sin2/1
  Square3/1 -> Sum8/2
  Sin4/1 -> Product5/2
  Constant5/1 -> Product3/1
  Constant7/1 -> Product5/1
  Product6/1 -> Sum7/1
  Product3/1 -> Sum6/2
  [th2] -> Sin4/1
  Product5/1 -> Sum7/2
  [th1] -> Sin5/1
  Sin3/1 -> Product4/2
  Constant8/1 -> Product6/1
  Sin5/1 -> Product6/2
  Sin2/1 -> Product3/2
  Sum6/1 -> Square2/1  "foot x position"
  Constant6/1 -> Product4/1
  Product4/1 -> Sum6/1
  Sum8/1 -> Square Root1/1
  [th1] -> Sin3/1
  Square Root1/1 -> current length/1  "current length"
  Bus Selector/1 -> Sum/1  "<knee_angle>"
  Bus Selector/2 -> Sum/2, [th1]  "<hip_angle>"
  measLeg/1 -> Bus Selector/1
  Sum/1 -> [th2]

== matlab function QuadrupedURDF/Subsystem/Cartesian -> Polar Jacobian ==
  data: joints_cartesian input; joints_polar output
function joints_polar = kinematics(joints_cartesian)

joints_polar = joints_cartesian;

end

== matlab function QuadrupedURDF/Subsystem/Polar -> Cartesian Jacobian ==
  data: joints_polar input; joints_cartesian output
function joints_cartesian = inv_kinematics(joints_polar)

joints_cartesian = joints_polar;

end

== stateflow chart QuadrupedURDF/Subsystem/SLIP Controller ==
  state Flight
  state Stance
  (default) -> Flight
  Stance -> Flight : [contacts(1) == 0]
  Flight -> Stance : [contacts(1) == 1]
  data: sf_internal_action_state_placeholder_data local double size=1 =0; sf_internal_action_state_placeholder_data local double size=1 =0

== stateflow chart QuadrupedURDF/Subsystem/Walking Gait ==
  note: WALKING GAIT
      | Step Order: FL-BR-FR-BL
      |
      | Switch states when step_time has elapsed; during switch reset timer,
      | set stepping
  state FL
  state BL
  state BR
  state FR
  (default) -> FL
  BL -> FL
  FL -> BR
  FR -> BL
  BR -> FR
